simulink model "untitled"  (Simulink 8.1)
settings: Solver=ode45  StartTime=0.0  StopTime=10.0  RelTol=1e-3
libraries: xbsIndex_r4 x498, dspsrcs4 x1
settings Model: Creator=spiro user  LastModifiedBy=spiro user
settings DataIOCC: SignalLoggingSaveFormat=Dataset
settings OptimizationCC: ExpressionDepthLimit=128
settings DebuggingCC: FcnCallInpInsideContextMsg=EnableAllAsError
settings GRTTargetCC: CombineOutputUpdateFcns=on  GRTInterface=off

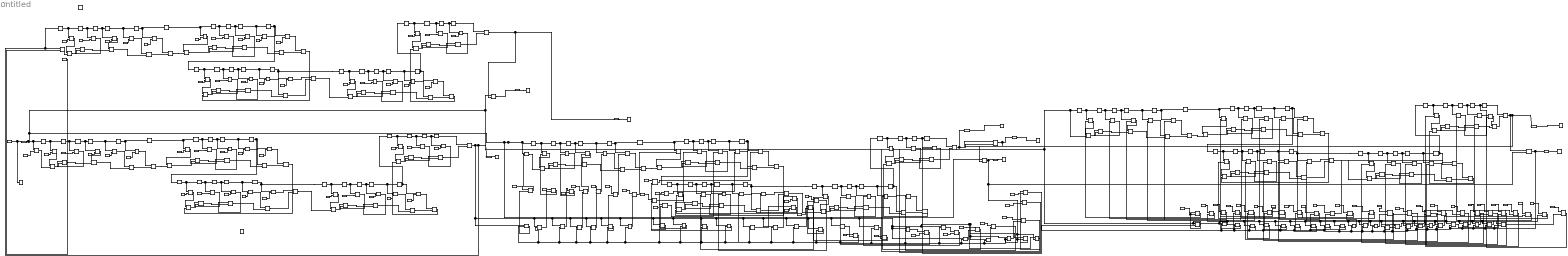
== system untitled ==
  " System Generator" : xbsIndex_r4/ System Generator  Tag=genX  xilinxfamily=artix7  part=xc7a200t  speed=-3  package=fbg676  synthesis_tool=XST  clock_wrapper=Clock Enables  directory=D:/xilinxsystemgeneratorusingaudionoise/firfiltersubmodule/netlist4  proj_type=Project Navigator  Synth_file=XST Defaults  Impl_file=ISE Defaults  testbench=off  simulink_period=1  sysclk_period=20  dcm_input_clock_period=10  incr_netlist=off  trim_vbits=Everywhere in SubSystem  dbl_ovrd=According to Block Masks  core_generation=According to Block Masks  run_coregen=off  deprecated_control=off  eval_field=0  block_type=sysgen
  AddSub : xbsIndex_r4/AddSub  mode=Subtraction  use_carryin=off  use_carryout=off  en=off  latency=0  precision=Full  arith_type=Unsigned  n_bits=16  bin_pt=14  quantization=Truncate  overflow=Wrap  dbl_ovrd=off  use_behavioral_HDL=off  hw_selection=Fabric  pipelined=off  block_type=addsub
  AddSub{1..25,27..96,98..125,130..151} (145 alike) : xbsIndex_r4/AddSub  mode=Addition  use_carryin=off  use_carryout=off  en=off  latency=0  precision=Full  arith_type=Unsigned  n_bits=16  bin_pt=14  quantization=Truncate  overflow=Wrap  dbl_ovrd=off  use_behavioral_HDL=off  hw_selection=Fabric  pipelined=off  block_type=addsub
  AddSub127 : xbsIndex_r4/AddSub  mode=Subtraction  use_carryin=off  use_carryout=off  en=off  latency=0  precision=Full  arith_type=Unsigned  n_bits=16  bin_pt=14  quantization=Truncate  overflow=Wrap  dbl_ovrd=off  use_behavioral_HDL=off  hw_selection=Fabric  pipelined=off  block_type=addsub
  AddSub26 : xbsIndex_r4/AddSub  mode=Addition  use_carryin=off  use_carryout=off  en=off  latency=0  precision=User Defined  arith_type=Unsigned  n_bits=16  bin_pt=14  quantization=Truncate  overflow=Wrap  dbl_ovrd=off  use_behavioral_HDL=off  hw_selection=Fabric  pipelined=off  block_type=addsub
  AddSub97 : xbsIndex_r4/AddSub  mode=Subtraction  use_carryin=off  use_carryout=off  en=off  latency=0  precision=Full  arith_type=Unsigned  n_bits=16  bin_pt=14  quantization=Truncate  overflow=Wrap  dbl_ovrd=off  use_behavioral_HDL=off  hw_selection=Fabric  pipelined=off  block_type=addsub
  Constant{,1,4..7,10..13,16..19,24..25,28..29,48..53,55..58,61..62,64..65,67..70} (36 alike) : xbsIndex_r4/Constant  const=1  gui_display_data_type=Fixed-point  arith_type=Signed (2's comp)  n_bits=16  bin_pt=14  preci_type=Double  exp_width=8  frac_width=24  explicit_period=off  period=1  equ=P=C  opselect=C  inp2=PCIN>>17  opr=+  inp1=P  carry=CIN  dbl_ovrd=off  block_type=constant
  Constant{2..3,8,14,20,26,54,59..60,63,66,71..95} (36 alike) : xbsIndex_r4/Constant  const=1  gui_display_data_type=Fixed-point  arith_type=Signed (2's comp)  n_bits=16  bin_pt=14  preci_type=Double  exp_width=8  frac_width=24  explicit_period=on  period=1  equ=P=C  opselect=C  inp2=PCIN>>17  opr=+  inp1=P  carry=CIN  dbl_ovrd=off  block_type=constant
  Constant{9,15,21..23,27,30..47} (24 alike) : xbsIndex_r4/Constant  const=1  gui_display_data_type=Fixed-point  arith_type=Signed (2's comp)  n_bits=16  bin_pt=14  preci_type=Single  exp_width=8  frac_width=24  explicit_period=off  period=1  equ=P=C  opselect=C  inp2=PCIN>>17  opr=+  inp1=P  carry=CIN  dbl_ovrd=off  block_type=constant
  Delay{,1..77,79..97} (97 alike) : xbsIndex_r4/Delay  rst=off  infoeditControl=Selection of Reset will increase slice count due to use of real FFs and instead of SRLs  en=off  latency=1  dbl_ovrd=off  reg_retiming=off  block_type=delay
  FDATool : xbsIndex_r4/FDATool  block_type=fdatool
      settings: infoedit=FDATool
  Gateway In : xbsIndex_r4/Gateway In  gui_display_data_type=Fixed-point  arith_type="Signed  (2's comp)"  n_bits=16  bin_pt=14  preci_type=Single  exp_width=8  frac_width=24  quantization="Round  (unbiased: +/- Inf)"  overflow=Saturate  period=1  dbl_ovrd=off  timing_constraint=None  locs_specified=off  LOCs={}  UseAsADC=off  ADCChannel='1'  inherit_from_input=off  hdl_port=on  block_type=gatewayin
  Gateway Out{,1..7} (8 alike) : xbsIndex_r4/Gateway Out  inherit_from_input=off  hdl_port=on  timing_constraint=None  locs_specified=off  LOCs={}  UseAsDAC=off  DACChannel='1'  block_type=gatewayout
  Mult{,1..7,9,11..13,15..27,29..41,43,45..48,72..73,75..87,89..95,120..121,123..135,137..143} (87 alike) : xbsIndex_r4/Mult  precision=User Defined  arith_type="Signed  (2's comp)"  n_bits=16  bin_pt=14  quantization=Truncate  overflow=Wrap  en=off  latency=3  dbl_ovrd=off  use_behavioral_HDL=off  opt=Speed  use_embedded=on  optimum_pipeline=off  pipeline=on  use_rpm=on  placement_style=Triangular  block_type=mult
  Mult{10,28,74,88,122,136} (6 alike) : xbsIndex_r4/Mult  precision=Full  arith_type="Signed  (2's comp)"  n_bits=16  bin_pt=14  quantization=Truncate  overflow=Wrap  en=off  latency=3  dbl_ovrd=off  use_behavioral_HDL=off  opt=Speed  use_embedded=on  optimum_pipeline=off  pipeline=on  use_rpm=on  placement_style=Triangular  block_type=mult
  Mult{8,14,42,44,49..71,96..119} (51 alike) : xbsIndex_r4/Mult  precision=User Defined  arith_type="Signed  (2's comp)"  n_bits=16  bin_pt=14  quantization=Truncate  overflow=Wrap  en=off  latency=1  dbl_ovrd=off  use_behavioral_HDL=off  opt=Speed  use_embedded=on  optimum_pipeline=off  pipeline=on  use_rpm=on  placement_style=Triangular  block_type=mult
  Resource Estimator : xbsIndex_r4/Resource Estimator  Tag=resEstTag  Slices=0  FFs=0  BRAMs=0  LUTs=0  IOBs=0  EBMs=0  TBUFs=0  xl_use_estimator_area=off  est_options=Estimate  block_type=resource_estimator
      settings: AttributesFormatString=Resource\nEstimator
  Signal From Workspace : dspsrcs4/Signal From Workspace  X=K  Ts=0.1  nsamps=1  OutputAfterFinalValue=Setting to zero  ignoreOrWarnInputAndFrameLengths=off
  Time Scope{,1..8} (9 alike) : TimeScope  DefaultConfigurationName=spbscopes.TimeScopeBlockCfg
      settings: CopyFcn=scopeextensions.ScopeBlock.callback(gcbh, 'onBlockCopy', gcbh);  DeleteFcn=scopeextensions.ScopeBlock.callback(gcbh, 'onBlockDelete');  PreSaveFcn=scopeextensions.ScopeBlock.callback(gcbh, 'onModelSave');  NameChangeFcn=scopeextensions.ScopeBlock.callback(gcbh, 'onBlockRename');  CloseFcn=scopeextensions.ScopeBlock.callback(gcbh, 'onBlockClose');  PreDeleteFcn=scopeextensions.ScopeBlock.callback(gcbh, 'onBlockPreDelete');
  wires:
  Constant3/1 -> Mult2/2
  Delay3/1 -> Mult/1, Delay2/1
  Mult2/1 -> AddSub3/2
  Delay/1 -> Mult1/1, Delay3/1
  Constant2/1 -> Mult1/2
  Mult1/1 -> AddSub3/1
  AddSub3/1 -> AddSub2/2
  Mult/1 -> AddSub2/1
  Constant/1 -> Mult3/2
  Delay2/1 -> Mult3/1, Delay1/1
  Delay1/1 -> Mult4/1, Delay4/1
  AddSub2/1 -> AddSub1/2
  Mult3/1 -> AddSub1/1
  AddSub1/1 -> AddSub4/2
  Constant1/1 -> Mult/2
  Constant4/1 -> Mult4/2
  Mult4/1 -> AddSub4/1
  Constant5/1 -> Mult5/2
  Mult5/1 -> AddSub5/1
  AddSub4/1 -> AddSub5/2
  Delay8/1 -> Mult6/1, Delay7/1
  Delay5/1 -> Delay8/1, Mult7/1
  Constant8/1 -> Mult7/2
  Mult7/1 -> AddSub8/1
  AddSub8/1 -> AddSub7/2
  Mult6/1 -> AddSub7/1
  Constant6/1 -> Mult9/2
  Delay7/1 -> Mult9/1, Delay6/1
  Delay6/1 -> Mult10/1, Delay9/1
  Delay4/1 -> Mult5/1, Delay5/1
  AddSub7/1 -> AddSub6/2
  Mult9/1 -> AddSub6/1
  AddSub6/1 -> AddSub9/2
  Constant7/1 -> Mult6/2
  Constant10/1 -> Mult10/2
  Mult10/1 -> AddSub9/1
  Constant11/1 -> Mult11/2
  Mult11/1 -> AddSub10/1
  AddSub9/1 -> AddSub10/2
  Delay13/1 -> Mult12/1, Delay12/1
  Delay10/1 -> Mult13/1, Delay13/1
  Constant14/1 -> Mult13/2
  Mult13/1 -> AddSub13/1
  AddSub13/1 -> AddSub12/2
  Mult12/1 -> AddSub12/1
  Constant12/1 -> Mult15/2
  Delay12/1 -> Mult15/1, Delay11/1
  Delay11/1 -> Mult16/1, Delay14/1
  Delay9/1 -> Delay10/1, Mult11/1
  AddSub12/1 -> AddSub11/2
  Mult15/1 -> AddSub11/1
  AddSub11/1 -> AddSub14/2
  Constant13/1 -> Mult12/2
  Constant16/1 -> Mult16/2
  Mult16/1 -> AddSub14/1
  Constant17/1 -> Mult17/2
  Mult17/1 -> AddSub15/1
  AddSub14/1 -> AddSub15/2
  Delay18/1 -> Mult18/1, Delay17/1
  Delay15/1 -> Mult19/1, Delay18/1
  Constant20/1 -> Mult19/2
  Mult19/1 -> AddSub18/1
  AddSub18/1 -> AddSub17/2
  Mult18/1 -> AddSub17/1
  Constant18/1 -> Mult21/2
  Delay17/1 -> Mult21/1, Delay16/1
  Delay16/1 -> AddSub19/1
  Delay24/1 -> Mult29/1, Delay15/1
  AddSub17/1 -> AddSub16/2
  Mult21/1 -> AddSub16/1
  Constant19/1 -> Mult18/2
  AddSub16/1 -> AddSub19/2
  Delay23/1 -> Mult24/1, Delay22/1
  AddSub15/1 -> AddSub23/2
  Delay20/1 -> Mult25/1, Delay23/1
  Constant26/1 -> Mult25/2
  Mult25/1 -> AddSub23/1
  AddSub23/1 -> AddSub22/2
  Mult24/1 -> AddSub22/1
  Constant24/1 -> Mult27/2
  Delay22/1 -> Mult27/1, Delay21/1
  Delay21/1 -> Mult28/1, Delay24/1
  Delay14/1 -> Delay20/1, Mult17/1
  AddSub22/1 -> AddSub21/2
  Mult27/1 -> AddSub21/1
  AddSub21/1 -> AddSub24/2
  Constant25/1 -> Mult24/2
  Constant28/1 -> Mult28/2
  Mult28/1 -> AddSub24/1
  Constant29/1 -> Mult29/2
  Mult29/1 -> AddSub25/1
  AddSub24/1 -> AddSub25/2
  AddSub5/1 -> AddSub8/2
  AddSub10/1 -> AddSub13/2
  AddSub25/1 -> AddSub18/2
  Gateway Out/1 -> Time Scope/1
  Delay41/1 -> Mult8/1, Delay35/1
  Mult35/1 -> AddSub42/2
  Delay19/1 -> Mult14/1, Delay41/1
  Mult14/1 -> AddSub42/1
  AddSub42/1 -> AddSub36/2
  Mult8/1 -> AddSub36/1
  Delay35/1 -> Mult42/1, Delay25/1
  Delay25/1 -> Mult43/1, Delay42/1
  AddSub36/1 -> AddSub20/2
  Mult42/1 -> AddSub20/1
  AddSub20/1 -> AddSub43/2
  Mult43/1 -> AddSub43/1
  Mult44/1 -> AddSub44/1
  AddSub43/1 -> AddSub44/2
  Delay46/1 -> Mult45/1, Delay45/1
  Delay43/1 -> Delay46/1, Mult46/1
  Mult46/1 -> AddSub47/1
  AddSub47/1 -> AddSub46/2
  Mult45/1 -> AddSub46/1
  Delay45/1 -> Mult47/1, Delay44/1
  Delay44/1 -> Mult20/1, Delay47/1
  Delay42/1 -> Mult44/1, Delay43/1
  AddSub46/1 -> AddSub45/2
  Mult47/1 -> AddSub45/1
  AddSub45/1 -> AddSub48/2
  Mult20/1 -> AddSub48/1
  Mult22/1 -> AddSub26/1
  AddSub48/1 -> AddSub26/2
  Delay29/1 -> Mult23/1, Delay28/1
  Delay26/1 -> Mult26/1, Delay29/1
  Mult26/1 -> AddSub29/1
  AddSub29/1 -> AddSub28/2
  Mult23/1 -> AddSub28/1
  Delay28/1 -> Mult30/1, Delay27/1
  Delay27/1 -> Mult31/1, Delay30/1
  Delay47/1 -> Delay26/1, Mult22/1
  AddSub28/1 -> AddSub27/2
  Mult30/1 -> AddSub27/1
  AddSub27/1 -> AddSub30/2
  Mult31/1 -> AddSub30/1
  Mult32/1 -> AddSub31/1
  AddSub30/1 -> AddSub31/2
  Delay34/1 -> Mult33/1, Delay33/1
  Delay31/1 -> Mult34/1, Delay34/1
  Mult34/1 -> AddSub34/1
  AddSub34/1 -> AddSub33/2
  Mult33/1 -> AddSub33/1
  Delay33/1 -> Mult36/1, Delay32/1
  Delay32/1 -> AddSub35/1
  Delay40/1 -> Mult41/1, Delay31/1
  AddSub33/1 -> AddSub32/2
  Mult36/1 -> AddSub32/1
  AddSub32/1 -> AddSub35/2
  Delay39/1 -> Mult37/1, Delay38/1
  AddSub31/1 -> AddSub39/2
  Delay36/1 -> Mult38/1, Delay39/1
  Mult38/1 -> AddSub39/1
  AddSub39/1 -> AddSub38/2
  Mult37/1 -> AddSub38/1
  Delay38/1 -> Mult39/1, Delay37/1
  Delay37/1 -> Mult40/1, Delay40/1
  Delay30/1 -> Delay36/1, Mult32/1
  AddSub38/1 -> AddSub37/2
  Mult39/1 -> AddSub37/1
  AddSub37/1 -> AddSub40/2
  Mult40/1 -> AddSub40/1
  Mult41/1 -> AddSub41/1
  AddSub40/1 -> AddSub41/2
  AddSub44/1 -> AddSub47/2
  AddSub26/1 -> AddSub29/2
  AddSub41/1 -> AddSub34/2
  Gateway Out1/1 -> Time Scope2/1
  Gateway Out2/1 -> Time Scope3/1
  Mult48/1 -> AddSub49/2
  Constant9/1 -> AddSub49/1
  AddSub49/1 -> Mult35/2
  Mult49/1 -> AddSub50/2
  AddSub50/1 -> Mult14/2
  Mult51/1 -> AddSub51/2
  Constant15/1 -> AddSub50/1
  Constant21/1 -> AddSub51/1
  AddSub51/1 -> Mult8/2
  Constant22/1 -> AddSub52/1
  Mult52/1 -> AddSub52/2
  AddSub52/1 -> Mult42/2
  Constant23/1 -> AddSub53/1
  Mult53/1 -> AddSub53/2
  AddSub53/1 -> Mult43/2
  Constant27/1 -> AddSub54/1
  Mult55/1 -> AddSub54/2
  AddSub54/1 -> Mult44/2
  Constant30/1 -> AddSub55/1
  Mult54/1 -> AddSub55/2
  AddSub55/1 -> Mult46/2
  Constant31/1 -> AddSub56/1
  Mult56/1 -> AddSub56/2
  AddSub56/1 -> Mult45/2
  Constant32/1 -> AddSub57/1
  Mult57/1 -> AddSub57/2
  AddSub57/1 -> Mult47/2
  Constant33/1 -> AddSub58/1
  Mult58/1 -> AddSub58/2
  AddSub58/1 -> Mult20/2
  Constant34/1 -> AddSub59/1
  Mult59/1 -> AddSub59/2
  AddSub59/1 -> Mult22/2
  Constant35/1 -> AddSub60/2
  Mult60/1 -> AddSub60/1
  AddSub60/1 -> Mult26/2
  Constant36/1 -> AddSub61/2
  Mult62/1 -> AddSub61/1
  AddSub61/1 -> Mult23/2
  Mult63/1 -> AddSub62/2
  Constant37/1 -> AddSub62/1
  AddSub62/1 -> Mult30/2
  Constant38/1 -> AddSub63/1
  Mult64/1 -> AddSub63/2
  AddSub63/1 -> Mult31/2
  Constant39/1 -> AddSub64/1
  Mult65/1 -> AddSub64/2
  AddSub64/1 -> Mult38/2
  Constant40/1 -> AddSub65/2
  Mult66/1 -> AddSub65/1
  AddSub65/1 -> Mult37/2
  Constant41/1 -> AddSub66/2
  Mult67/1 -> AddSub66/1
  AddSub66/1 -> Mult39/2
  Mult68/1 -> AddSub67/2
  Constant42/1 -> AddSub67/1
  AddSub67/1 -> Mult40/2
  Constant43/1 -> AddSub68/1
  Mult69/1 -> AddSub68/2
  AddSub68/1 -> Mult41/2
  Constant44/1 -> AddSub69/1
  Mult70/1 -> AddSub69/2
  AddSub69/1 -> Mult34/2
  Constant45/1 -> AddSub70/2
  Mult50/1 -> AddSub71/1
  Mult71/1 -> AddSub70/1
  AddSub70/1 -> Mult33/2
  Constant46/1 -> AddSub71/2
  AddSub71/1 -> Mult36/2
  Constant47/1 -> AddSub72/2
  Mult61/1 -> AddSub72/1
  AddSub72/1 -> Mult32/2
  Delay65/1 -> Mult72/1, Delay59/1
  Delay48/1 -> Mult73/1, Delay65/1
  Mult73/1 -> AddSub90/1
  AddSub90/1 -> AddSub84/2
  Mult72/1 -> AddSub84/1
  Delay59/1 -> Mult90/1, Delay49/1
  Delay49/1 -> Mult91/1, Delay66/1
  AddSub84/1 -> AddSub73/2
  Mult90/1 -> AddSub73/1
  AddSub73/1 -> AddSub91/2
  Mult91/1 -> AddSub91/1
  Mult92/1 -> AddSub92/1
  AddSub91/1 -> AddSub92/2
  Delay70/1 -> Mult93/1, Delay69/1
  Delay67/1 -> Delay70/1, Mult94/1
  Mult94/1 -> AddSub95/1
  AddSub95/1 -> AddSub94/2
  Mult93/1 -> AddSub94/1
  Delay69/1 -> Mult95/1, Delay68/1
  Delay68/1 -> Mult74/1, Delay71/1
  Delay66/1 -> Mult92/1, Delay67/1
  AddSub94/1 -> AddSub93/2
  Mult95/1 -> AddSub93/1
  AddSub93/1 -> AddSub96/2
  AddSub104/1 -> Mult93/2
  Mult74/1 -> AddSub96/1
  Mult75/1 -> AddSub74/1
  AddSub96/1 -> AddSub74/2
  Delay53/1 -> Mult76/1, Delay52/1
  Delay50/1 -> Mult77/1, Delay53/1
  Mult77/1 -> AddSub77/1
  AddSub77/1 -> AddSub76/2
  Mult76/1 -> AddSub76/1
  Delay52/1 -> Mult78/1, Delay51/1
  Delay51/1 -> Mult79/1, Delay54/1
  Delay71/1 -> Delay50/1, Mult75/1
  AddSub76/1 -> AddSub75/2
  Mult78/1 -> AddSub75/1
  AddSub75/1 -> AddSub78/2
  Mult79/1 -> AddSub78/1
  Mult80/1 -> AddSub79/1
  AddSub78/1 -> AddSub79/2
  Delay58/1 -> Mult81/1, Delay57/1
  Delay55/1 -> Mult82/1, Delay58/1
  Mult82/1 -> AddSub82/1
  AddSub82/1 -> AddSub81/2
  Mult81/1 -> AddSub81/1
  Delay57/1 -> Mult84/1, Delay56/1
  Delay64/1 -> Mult89/1, Delay55/1
  AddSub81/1 -> AddSub80/2
  Mult84/1 -> AddSub80/1
  Delay63/1 -> Mult85/1, Delay62/1
  AddSub79/1 -> AddSub87/2
  Delay60/1 -> Mult86/1, Delay63/1
  Mult86/1 -> AddSub87/1
  AddSub87/1 -> AddSub86/2
  Mult85/1 -> AddSub86/1
  Delay62/1 -> Mult87/1, Delay61/1
  Delay61/1 -> Mult88/1, Delay64/1
  Delay54/1 -> Delay60/1, Mult80/1
  AddSub86/1 -> AddSub85/2
  Mult87/1 -> AddSub85/1
  AddSub85/1 -> AddSub88/2
  Mult88/1 -> AddSub88/1
  AddSub107/1 -> Mult89/2
  Mult89/1 -> AddSub89/1
  AddSub88/1 -> AddSub89/2
  AddSub92/1 -> AddSub95/2
  AddSub74/1 -> AddSub77/2
  AddSub89/1 -> AddSub82/2
  Gateway Out4/1 -> Time Scope5/1
  Gateway Out5/1 -> Time Scope6/1
  AddSub97/1 -> Mult97/2, Mult99/2, Mult101/2, Mult102/2, Mult103/2, Mult119/2, Mult118/2, Mult117/2, Mult116/2, Mult115/2, Mult114/2, Mult113/2, Mult112/2, Mult111/2, Mult110/2, Mult109/2, Mult108/2, Mult107/2, Mult106/2, Mult105/2, Mult104/2, Mult100/2, Mult98/2, Mult96/2, Gateway Out5/1
  Mult96/1 -> AddSub121/2
  Mult97/1 -> AddSub120/2
  Mult98/1 -> AddSub119/2
  Mult99/1 -> AddSub118/2
  Mult100/1 -> AddSub117/2
  Mult101/1 -> AddSub116/2
  Mult102/1 -> AddSub115/2
  Mult103/1 -> AddSub114/2
  Mult104/1 -> AddSub113/2
  Mult105/1 -> AddSub112/2
  Mult106/1 -> AddSub111/2
  Mult107/1 -> AddSub110/2
  Mult108/1 -> AddSub109/2
  Mult109/1 -> AddSub108/2
  Mult110/1 -> AddSub107/2
  Mult111/1 -> AddSub106/2
  Mult112/1 -> AddSub105/2
  Mult113/1 -> AddSub104/2
  Mult114/1 -> AddSub103/2
  Mult115/1 -> AddSub102/2
  Mult116/1 -> AddSub101/2
  Mult117/1 -> AddSub100/2
  Mult118/1 -> AddSub99/2
  Mult119/1 -> AddSub98/2
  Constant72/1 -> AddSub98/1
  Constant73/1 -> AddSub99/1
  Constant74/1 -> AddSub100/1
  Constant75/1 -> AddSub101/1
  Constant76/1 -> AddSub102/1
  Constant77/1 -> AddSub103/1
  Constant78/1 -> AddSub104/1
  Constant79/1 -> AddSub105/1
  Constant80/1 -> AddSub106/1
  Constant81/1 -> AddSub107/1
  Constant82/1 -> AddSub108/1
  Constant83/1 -> AddSub109/1
  Constant84/1 -> AddSub110/1
  Constant85/1 -> AddSub111/1
  Constant86/1 -> AddSub112/1
  Constant87/1 -> AddSub113/1
  Constant88/1 -> AddSub114/1
  Constant89/1 -> AddSub115/1
  Constant90/1 -> AddSub116/1
  Constant91/1 -> AddSub117/1
  Constant92/1 -> AddSub118/1
  Constant93/1 -> AddSub119/1
  Constant94/1 -> AddSub120/1
  Constant95/1 -> AddSub121/1
  AddSub98/1 -> Mult73/2
  AddSub99/1 -> Mult72/2
  AddSub100/1 -> Mult90/2
  AddSub101/1 -> Mult91/2
  AddSub102/1 -> Mult92/2
  AddSub103/1 -> Mult94/2
  AddSub105/1 -> Mult95/2
  AddSub106/1 -> Mult74/2
  AddSub108/1 -> Mult75/2
  AddSub109/1 -> Mult77/2
  AddSub110/1 -> Mult76/2
  AddSub111/1 -> Mult78/2
  AddSub112/1 -> Mult79/2
  AddSub113/1 -> Mult80/2
  AddSub114/1 -> Mult86/2
  AddSub115/1 -> Mult85/2
  AddSub116/1 -> Mult87/2
  AddSub117/1 -> Mult88/2
  AddSub118/1 -> Mult82/2
  AddSub119/1 -> Mult81/2
  AddSub120/1 -> Mult84/2
  Delay56/1 -> Mult83/1, Delay72/1
  AddSub80/1 -> AddSub122/2
  Mult83/1 -> AddSub122/1
  AddSub122/1 -> AddSub83/2
  Delay72/1 -> AddSub83/1
  AddSub121/1 -> Mult83/2
  AddSub35/1 -> Gateway Out7/1, AddSub123/2
  AddSub83/1 -> AddSub123/1, Gateway Out4/1, AddSub97/1
  Gateway Out7/1 -> Time Scope7/1
  Signal From Workspace/1 -> Time Scope1/1, Gateway In/1
  Gateway Out6/1 -> Time Scope8/1
  AddSub123/1 -> AddSub/2, Gateway Out2/1
  Delay91/1 -> Mult120/1, Delay85/1
  Mult131/1 -> AddSub145/2
  Delay73/1 -> Mult121/1, Delay91/1
  Constant59/1 -> Mult121/2
  Mult121/1 -> AddSub145/1
  AddSub145/1 -> AddSub139/2
  Mult120/1 -> AddSub139/1
  Constant48/1 -> Mult138/2
  Delay85/1 -> Mult138/1, Delay74/1
  Delay74/1 -> Mult139/1, Delay92/1
  AddSub139/1 -> AddSub124/2
  Mult138/1 -> AddSub124/1
  AddSub124/1 -> AddSub146/2
  Constant49/1 -> Mult120/2
  Constant67/1 -> Mult139/2
  Mult139/1 -> AddSub146/1
  Constant68/1 -> Mult140/2
  Mult140/1 -> AddSub147/1
  AddSub146/1 -> AddSub147/2
  Delay96/1 -> Mult141/1, Delay95/1
  Delay93/1 -> Delay96/1, Mult142/1
  Constant71/1 -> Mult142/2
  Mult142/1 -> AddSub150/1
  AddSub150/1 -> AddSub149/2
  Mult141/1 -> AddSub149/1
  Constant69/1 -> Mult143/2
  Delay95/1 -> Mult143/1, Delay94/1
  Delay94/1 -> Mult122/1, Delay97/1
  Delay92/1 -> Mult140/1, Delay93/1
  AddSub149/1 -> AddSub148/2
  Mult143/1 -> AddSub148/1
  AddSub148/1 -> AddSub151/2
  Constant70/1 -> Mult141/2
  Constant50/1 -> Mult122/2
  Mult122/1 -> AddSub151/1
  Constant51/1 -> Mult123/2
  Mult123/1 -> AddSub125/1
  AddSub151/1 -> AddSub125/2
  Delay79/1 -> Mult124/1, Delay77/1
  Delay75/1 -> Mult125/1, Delay79/1
  Constant54/1 -> Mult125/2
  Mult125/1 -> AddSub132/1
  AddSub132/1 -> AddSub131/2
  Mult124/1 -> AddSub131/1
  Constant52/1 -> Mult126/2
  Delay77/1 -> Mult126/1, Delay76/1
  Delay76/1 -> Mult127/1, Delay80/1
  Delay97/1 -> Delay75/1, Mult123/1
  AddSub131/1 -> AddSub130/2
  Mult126/1 -> AddSub130/1
  AddSub130/1 -> AddSub133/2
  Constant53/1 -> Mult124/2
  Constant55/1 -> Mult127/2
  Mult127/1 -> AddSub133/1
  Constant56/1 -> Mult128/2
  Mult128/1 -> AddSub134/1
  AddSub133/1 -> AddSub134/2
  Constant60/1 -> Mult130/2
  Mult130/1 -> AddSub137/1
  AddSub137/1 -> AddSub136/2
  Mult129/1 -> AddSub136/1
  Constant57/1 -> Mult132/2
  Delay82/1 -> AddSub138/1
  Delay90/1 -> Mult137/1, Delay81/1
  AddSub136/1 -> AddSub135/2
  Mult132/1 -> AddSub135/1
  Constant58/1 -> Mult129/2
  AddSub135/1 -> AddSub138/2
  Delay89/1 -> Mult133/1, Delay88/1
  AddSub134/1 -> AddSub142/2
  Delay86/1 -> Mult134/1, Delay89/1
  Constant63/1 -> Mult134/2
  Mult134/1 -> AddSub142/1
  AddSub142/1 -> AddSub141/2
  Mult133/1 -> AddSub141/1
  Constant61/1 -> Mult135/2
  Delay88/1 -> Mult135/1, Delay87/1
  Delay87/1 -> Mult136/1, Delay90/1
  Delay80/1 -> Delay86/1, Mult128/1
  AddSub141/1 -> AddSub140/2
  Mult135/1 -> AddSub140/1
  AddSub140/1 -> AddSub143/2
  Constant62/1 -> Mult133/2
  Constant64/1 -> Mult136/2
  Mult136/1 -> AddSub143/1
  Constant65/1 -> Mult137/2
  Mult137/1 -> AddSub144/1
  AddSub143/1 -> AddSub144/2
  AddSub147/1 -> AddSub150/2
  AddSub125/1 -> AddSub132/2
  AddSub144/1 -> AddSub137/2
  Delay84/1 -> Mult129/1, Delay83/1
  Delay81/1 -> Mult130/1, Delay84/1
  Delay83/1 -> Mult132/1, Delay82/1
  AddSub/1 -> Gateway Out1/1, AddSub97/2, Mult50/2, Mult70/2, Mult69/2, Mult68/2, Mult67/2, Mult66/2, Mult65/2, Mult64/2, Mult63/2, Mult62/2, Mult61/2, Mult60/2, Mult59/2, Mult58/2, Mult57/2, Mult56/2, Mult54/2, Mult55/2, Mult53/2, Mult52/2, Mult51/2, Mult49/2, Mult48/2, Mult71/2
  Constant66/1 -> Mult131/2
  Gateway Out3/1 -> Time Scope4/1
  AddSub127/1 -> Gateway Out3/1
  AddSub138/1 -> AddSub127/2, Gateway Out6/1
  Gateway In/1 -> AddSub127/1, Delay48/1, AddSub90/2, Mult99/1, Mult98/1, Mult97/1, Mult96/1, Mult100/1, Mult101/1, Mult102/1, Mult103/1, Mult104/1, Mult106/1, Mult105/1, Mult107/1, Mult108/1, Mult109/1, Mult110/1, Mult111/1, Mult112/1, Mult113/1, Mult114/1, Mult115/1, Mult116/1, Mult117/1, Mult118/1, Mult119/1, AddSub/1, Mult35/1, Delay19/1, Mult2/1, Delay/1
  AddSub19/1 -> Mult48/1, Mult49/1, Mult51/1, Mult52/1, Mult53/1, Mult55/1, Mult54/1, Mult56/1, Mult57/1, Mult58/1, Mult59/1, Mult60/1, Mult61/1, Mult62/1, Mult63/1, Mult64/1, Mult65/1, Mult68/1, Mult66/1, Mult67/1, Mult50/1, Mult71/1, Mult70/1, Mult69/1, Delay73/1, Mult131/1, Gateway Out/1
